simulink model "ASM_Traffic_V2X_Complete_Model_2"  (R2019a)
settings: Solver=ode1  StartTime=SIM.tstart.v  StopTime=Inf  FixedStep=SIM.StepSize.v  RelTol=1e-3
PostLoadFcn:
  | if any(exist('dsrtsu_mdlpostloadfcn', 'file') ~= 0), dsrtsu_mdlpostloadfcn('Execute', bdroot); end
  | try, asm_mdl_postloadfcn(bdroot, 'UpdateModel', 2200); catch, disp(lasterr); end,
undefined symbols (not defined in the file): _SensorPnts_1, _SensorPnts_13, _SensorPnts_17, _SensorPnts_21, _SensorPnts_25, _SensorPnts_29, _SensorPnts_33, _SensorPnts_37, _SensorPnts_41, _SensorPnts_45, _SensorPnts_49, _SensorPnts_5, _SensorPnts_53, _SensorPnts_57, _SensorPnts_9, _to_, CPT, G5A, ITS, MDL, rad, s_to_rpm, SIM
libraries: simulink x169, ASM_VehicleDynamics_lib x126, ASM_Traffic_lib x83, ASM_Utils_lib x49, mdbs x45, ASM_Environment_lib x17, dspindex x12, dsaV2xLibraryAux x10, dsmpblib x6, dsaV2xAsn1Library x4, dsaV2xLibrary x4, ASM_BrakeHydraulics_lib x4
(part 4 of 36)

== system ASM_Traffic_V2X_Complete_Model_2/MDL/MDL_In/Ctrl_ChangeOverValve_1[0_1] ==
  SoftECU : Inport
  RealECU : Inport  Port=2
  Const_Ctrl_ChangeOverValve_1[0_1] : Constant  Value=0
  MultiPortSwitch : MultiPortSwitch  SaturateOnIntegerOverflow=on  InputSameDT=on
  Sw_Ctrl_ChangeOverValve_1[1SoftECU|2RealECU|3Const] : Constant  Value=CPT.MDL_SW.Sw_Ctrl_ChangeOverValve_1.v
  Ctrl_ChangeOverValve_1[0_1] : Outport
  wires:
  MultiPortSwitch/1 -> Ctrl_ChangeOverValve_1[0_1]/1
  Const_Ctrl_ChangeOverValve_1[0_1]/1 -> MultiPortSwitch/4
  RealECU/1 -> MultiPortSwitch/3
  SoftECU/1 -> MultiPortSwitch/2
  Sw_Ctrl_ChangeOverValve_1[1SoftECU|2RealECU|3Const]/1 -> MultiPortSwitch/1

== system ASM_Traffic_V2X_Complete_Model_2/MDL/MDL_In/Ctrl_ChangeOverValve_2[0_1] ==
  SoftECU : Inport
  RealECU : Inport  Port=2
  Const_Ctrl_ChangeOverValve_2[0_1] : Constant  Value=0
  MultiPortSwitch : MultiPortSwitch  SaturateOnIntegerOverflow=on  InputSameDT=on
  Sw_Ctrl_ChangeOverValve_2[1SoftECU|2RealECU|3Const] : Constant  Value=CPT.MDL_SW.Sw_Ctrl_ChangeOverValve_2.v
  Ctrl_ChangeOverValve_2[0_1] : Outport
  wires:
  Sw_Ctrl_ChangeOverValve_2[1SoftECU|2RealECU|3Const]/1 -> MultiPortSwitch/1
  SoftECU/1 -> MultiPortSwitch/2
  RealECU/1 -> MultiPortSwitch/3
  Const_Ctrl_ChangeOverValve_2[0_1]/1 -> MultiPortSwitch/4
  MultiPortSwitch/1 -> Ctrl_ChangeOverValve_2[0_1]/1

== system ASM_Traffic_V2X_Complete_Model_2/MDL/MDL_In/Ctrl_Clutch_4WD[%] ==
  SoftECU : Inport
  RealECU : Inport  Port=2
  Const_Ctrl_Clutch_4WD[%] : Constant  Value=0
  MultiPortSwitch : MultiPortSwitch  SaturateOnIntegerOverflow=on  InputSameDT=on
  Sw_Clutch_4WD[1SoftECU|2RealECU|3Const] : Constant  Value=CPT.MDL_SW.Sw_Clutch_4WD.v
  Ctrl_Clutch_4WD[%] : Outport
  wires:
  Sw_Clutch_4WD[1SoftECU|2RealECU|3Const]/1 -> MultiPortSwitch/1
  SoftECU/1 -> MultiPortSwitch/2
  RealECU/1 -> MultiPortSwitch/3
  Const_Ctrl_Clutch_4WD[%]/1 -> MultiPortSwitch/4
  MultiPortSwitch/1 -> Ctrl_Clutch_4WD[%]/1

== system ASM_Traffic_V2X_Complete_Model_2/MDL/MDL_In/Ctrl_FrontDiff[%] ==
  SoftECU : Inport
  RealECU : Inport  Port=2
  Const_Ctrl_FrontDiff[%] : Constant  Value=0
  MultiPortSwitch : MultiPortSwitch  SaturateOnIntegerOverflow=on  InputSameDT=on
  Sw_Ctrl_FrontDiff[1SoftECU|2RealECU|3Const] : Constant  Value=CPT.MDL_SW.Sw_Ctrl_FrontDiff.v
  Ctrl_FrontDiff[%] : Outport
  wires:
  Sw_Ctrl_FrontDiff[1SoftECU|2RealECU|3Const]/1 -> MultiPortSwitch/1
  SoftECU/1 -> MultiPortSwitch/2
  RealECU/1 -> MultiPortSwitch/3
  Const_Ctrl_FrontDiff[%]/1 -> MultiPortSwitch/4
  MultiPortSwitch/1 -> Ctrl_FrontDiff[%]/1

== system ASM_Traffic_V2X_Complete_Model_2/MDL/MDL_In/Ctrl_HydPump[0_1] ==
  SoftECU : Inport
  RealECU : Inport  Port=2
  Const_Ctrl_HydPump[0_1] : Constant  Value=0
  MultiPortSwitch : MultiPortSwitch  SaturateOnIntegerOverflow=on  InputSameDT=on
  Sw_Ctrl_HydPump[1SoftECU|2RealECU|3Const] : Constant  Value=CPT.MDL_SW.Sw_Ctrl_HydPump.v
  Ctrl_HydPump[0_1] : Outport
  wires:
  Sw_Ctrl_HydPump[1SoftECU|2RealECU|3Const]/1 -> MultiPortSwitch/1
  SoftECU/1 -> MultiPortSwitch/2
  RealECU/1 -> MultiPortSwitch/3
  Const_Ctrl_HydPump[0_1]/1 -> MultiPortSwitch/4
  MultiPortSwitch/1 -> Ctrl_HydPump[0_1]/1

== system ASM_Traffic_V2X_Complete_Model_2/MDL/MDL_In/Ctrl_InletValve_FL[0_1] ==
  SoftECU : Inport
  RealECU : Inport  Port=2
  Const_Ctrl_InletValve_FL[0_1] : Constant  Value=0
  MultiPortSwitch : MultiPortSwitch  SaturateOnIntegerOverflow=on  InputSameDT=on
  Sw_Ctrl_InletValve_FL[1SoftECU|2RealECU|3Const] : Constant  Value=CPT.MDL_SW.Sw_Ctrl_InletValve_FL.v
  Ctrl_InletValve_FL[0_1] : Outport
  wires:
  Sw_Ctrl_InletValve_FL[1SoftECU|2RealECU|3Const]/1 -> MultiPortSwitch/1
  SoftECU/1 -> MultiPortSwitch/2
  RealECU/1 -> MultiPortSwitch/3
  Const_Ctrl_InletValve_FL[0_1]/1 -> MultiPortSwitch/4
  MultiPortSwitch/1 -> Ctrl_InletValve_FL[0_1]/1

== system ASM_Traffic_V2X_Complete_Model_2/MDL/MDL_In/Ctrl_InletValve_FR[0_1] ==
  SoftECU : Inport
  RealECU : Inport  Port=2
  Const_Ctrl_InletValve_FR[0_1] : Constant  Value=0
  MultiPortSwitch : MultiPortSwitch  SaturateOnIntegerOverflow=on  InputSameDT=on
  Sw_Ctrl_InletValve_FR[1SoftECU|2RealECU|3Const] : Constant  Value=CPT.MDL_SW.Sw_Ctrl_InletValve_FR.v
  Ctrl_InletValve_FR[0_1] : Outport
  wires:
  MultiPortSwitch/1 -> Ctrl_InletValve_FR[0_1]/1
  Const_Ctrl_InletValve_FR[0_1]/1 -> MultiPortSwitch/4
  RealECU/1 -> MultiPortSwitch/3
  SoftECU/1 -> MultiPortSwitch/2
  Sw_Ctrl_InletValve_FR[1SoftECU|2RealECU|3Const]/1 -> MultiPortSwitch/1

== system ASM_Traffic_V2X_Complete_Model_2/MDL/MDL_In/Ctrl_InletValve_RL[0_1] ==
  SoftECU : Inport
  RealECU : Inport  Port=2
  Const_Ctrl_InletValve_RL[0_1] : Constant  Value=0
  MultiPortSwitch : MultiPortSwitch  SaturateOnIntegerOverflow=on  InputSameDT=on
  Sw_Ctrl_InletValve_RL[1SoftECU|2RealECU|3Const] : Constant  Value=CPT.MDL_SW.Sw_Ctrl_InletValve_RL.v
  Ctrl_InletValve_RL[0_1] : Outport
  wires:
  MultiPortSwitch/1 -> Ctrl_InletValve_RL[0_1]/1
  Const_Ctrl_InletValve_RL[0_1]/1 -> MultiPortSwitch/4
  RealECU/1 -> MultiPortSwitch/3
  SoftECU/1 -> MultiPortSwitch/2
  Sw_Ctrl_InletValve_RL[1SoftECU|2RealECU|3Const]/1 -> MultiPortSwitch/1

== system ASM_Traffic_V2X_Complete_Model_2/MDL/MDL_In/Ctrl_InletValve_RR[0_1] ==
  SoftECU : Inport
  RealECU : Inport  Port=2
  Const_Ctrl_InletValve_RR[0_1] : Constant  Value=0
  MultiPortSwitch : MultiPortSwitch  SaturateOnIntegerOverflow=on  InputSameDT=on
  Sw_Ctrl_InletValve_RR[1SoftECU|2RealECU|3Const] : Constant  Value=CPT.MDL_SW.Sw_Ctrl_InletValve_RR.v
  Ctrl_InletValve_RR[0_1] : Outport
  wires:
  Sw_Ctrl_InletValve_RR[1SoftECU|2RealECU|3Const]/1 -> MultiPortSwitch/1
  SoftECU/1 -> MultiPortSwitch/2
  RealECU/1 -> MultiPortSwitch/3
  Const_Ctrl_InletValve_RR[0_1]/1 -> MultiPortSwitch/4
  MultiPortSwitch/1 -> Ctrl_InletValve_RR[0_1]/1

== system ASM_Traffic_V2X_Complete_Model_2/MDL/MDL_In/Ctrl_Lockup_Clutch[%] ==
  SoftECU : Inport
  RealECU : Inport  Port=2
  Const_Ctrl_Lockup_Clutch[%] : Constant  Value=0
  MultiPortSwitch : MultiPortSwitch  SaturateOnIntegerOverflow=on  InputSameDT=on
  Sw_Ctrl_Lockup_Clutch[1SoftECU|2RealECU|3Const] : Constant  Value=CPT.MDL_SW.Sw_Ctrl_Lockup_Clutch.v
  Ctrl_Lockup_Clutch[%] : Outport
  wires:
  Sw_Ctrl_Lockup_Clutch[1SoftECU|2RealECU|3Const]/1 -> MultiPortSwitch/1
  SoftECU/1 -> MultiPortSwitch/2
  RealECU/1 -> MultiPortSwitch/3
  Const_Ctrl_Lockup_Clutch[%]/1 -> MultiPortSwitch/4
  MultiPortSwitch/1 -> Ctrl_Lockup_Clutch[%]/1

== system ASM_Traffic_V2X_Complete_Model_2/MDL/MDL_In/Ctrl_OutletValve_FL[0_1] ==
  SoftECU : Inport
  RealECU : Inport  Port=2
  Const_Ctrl_OutletValve_FL[0_1] : Constant  Value=0
  MultiPortSwitch : MultiPortSwitch  SaturateOnIntegerOverflow=on  InputSameDT=on
  Sw_Ctrl_OutletValve_FL[1SoftECU|2RealECU|3Const] : Constant  Value=CPT.MDL_SW.Sw_Ctrl_OutletValve_FL.v
  Ctrl_OutletValve_FL[0_1] : Outport
  wires:
  Sw_Ctrl_OutletValve_FL[1SoftECU|2RealECU|3Const]/1 -> MultiPortSwitch/1
  SoftECU/1 -> MultiPortSwitch/2
  RealECU/1 -> MultiPortSwitch/3
  Const_Ctrl_OutletValve_FL[0_1]/1 -> MultiPortSwitch/4
  MultiPortSwitch/1 -> Ctrl_OutletValve_FL[0_1]/1

== system ASM_Traffic_V2X_Complete_Model_2/MDL/MDL_In/Ctrl_OutletValve_FR[0_1] ==
  SoftECU : Inport
  RealECU : Inport  Port=2
  Const_Ctrl_OutletValve_FR[0_1] : Constant  Value=0
  MultiPortSwitch : MultiPortSwitch  SaturateOnIntegerOverflow=on  InputSameDT=on
  Sw_Ctrl_OutletValve_FR[1SoftECU|2RealECU|3Const] : Constant  Value=CPT.MDL_SW.Sw_Ctrl_OutletValve_FR.v
  Ctrl_OutletValve_FR[0_1] : Outport
  wires:
  MultiPortSwitch/1 -> Ctrl_OutletValve_FR[0_1]/1
  Const_Ctrl_OutletValve_FR[0_1]/1 -> MultiPortSwitch/4
  RealECU/1 -> MultiPortSwitch/3
  SoftECU/1 -> MultiPortSwitch/2
  Sw_Ctrl_OutletValve_FR[1SoftECU|2RealECU|3Const]/1 -> MultiPortSwitch/1

== system ASM_Traffic_V2X_Complete_Model_2/MDL/MDL_In/Ctrl_OutletValve_RL[0_1] ==
  SoftECU : Inport
  RealECU : Inport  Port=2
  Const_Ctrl_OutletValve_RL[0_1] : Constant  Value=0
  MultiPortSwitch : MultiPortSwitch  SaturateOnIntegerOverflow=on  InputSameDT=on
  Sw_Ctrl_OutletValve_RL[1SoftECU|2RealECU|3Const] : Constant  Value=CPT.MDL_SW.Sw_Ctrl_OutletValve_RL.v
  Ctrl_OutletValve_RL[0_1] : Outport
  wires:
  MultiPortSwitch/1 -> Ctrl_OutletValve_RL[0_1]/1
  Const_Ctrl_OutletValve_RL[0_1]/1 -> MultiPortSwitch/4
  RealECU/1 -> MultiPortSwitch/3
  SoftECU/1 -> MultiPortSwitch/2
  Sw_Ctrl_OutletValve_RL[1SoftECU|2RealECU|3Const]/1 -> MultiPortSwitch/1

== system ASM_Traffic_V2X_Complete_Model_2/MDL/MDL_In/Ctrl_OutletValve_RR[0_1] ==
  SoftECU : Inport
  RealECU : Inport  Port=2
  Const_Ctrl_OutletValve_RR[0_1] : Constant  Value=0
  MultiPortSwitch : MultiPortSwitch  SaturateOnIntegerOverflow=on  InputSameDT=on
  Sw_Ctrl_OutletValve_RR[1SoftECU|2RealECU|3Const] : Constant  Value=CPT.MDL_SW.Sw_Ctrl_OutletValve_RR.v
  Ctrl_OutletValve_RR[0_1] : Outport
  wires:
  Sw_Ctrl_OutletValve_RR[1SoftECU|2RealECU|3Const]/1 -> MultiPortSwitch/1
  SoftECU/1 -> MultiPortSwitch/2
  RealECU/1 -> MultiPortSwitch/3
  Const_Ctrl_OutletValve_RR[0_1]/1 -> MultiPortSwitch/4
  MultiPortSwitch/1 -> Ctrl_OutletValve_RR[0_1]/1

== system ASM_Traffic_V2X_Complete_Model_2/MDL/MDL_In/Ctrl_Parking_Pawl[0|1] ==
  SoftECU : Inport
  RealECU : Inport  Port=2
  Const_Park_Lock[0|1] : Constant  Value=0
  MultiPortSwitch : MultiPortSwitch  SaturateOnIntegerOverflow=on  InputSameDT=on
  Sw_Parking_Pawl[1SoftECU|2RealECU|3Const] : Constant  Value=CPT.MDL_SW.Sw_Parking_Pawl.v
  Ctrl_Parking_Pawl[0|1] : Outport
  wires:
  Sw_Parking_Pawl[1SoftECU|2RealECU|3Const]/1 -> MultiPortSwitch/1
  SoftECU/1 -> MultiPortSwitch/2
  RealECU/1 -> MultiPortSwitch/3
  Const_Park_Lock[0|1]/1 -> MultiPortSwitch/4
  MultiPortSwitch/1 -> Ctrl_Parking_Pawl[0|1]/1

== system ASM_Traffic_V2X_Complete_Model_2/MDL/MDL_In/Ctrl_PreChargeValve_1[0_1] ==
  SoftECU : Inport
  RealECU : Inport  Port=2
  Const_Ctrl_PreChargeValve_1[0_1] : Constant  Value=0
  MultiPortSwitch : MultiPortSwitch  SaturateOnIntegerOverflow=on  InputSameDT=on
  Sw_Ctrl_PreChargeValve_1[1SoftECU|2RealECU|3Const] : Constant  Value=CPT.MDL_SW.Sw_Ctrl_PreChargeValve_1.v
  Ctrl_PreChargeValve_1[0_1] : Outport
  wires:
  Sw_Ctrl_PreChargeValve_1[1SoftECU|2RealECU|3Const]/1 -> MultiPortSwitch/1
  SoftECU/1 -> MultiPortSwitch/2
  RealECU/1 -> MultiPortSwitch/3
  Const_Ctrl_PreChargeValve_1[0_1]/1 -> MultiPortSwitch/4
  MultiPortSwitch/1 -> Ctrl_PreChargeValve_1[0_1]/1

== system ASM_Traffic_V2X_Complete_Model_2/MDL/MDL_In/Ctrl_PreChargeValve_2[0_1] ==
  SoftECU : Inport
  RealECU : Inport  Port=2
  Const_Ctrl_PreChargeValve_2[0_1] : Constant  Value=0
  MultiPortSwitch : MultiPortSwitch  SaturateOnIntegerOverflow=on  InputSameDT=on
  Sw_Ctrl_PreChargeValve_2[1SoftECU|2RealECU|3Const] : Constant  Value=CPT.MDL_SW.Sw_Ctrl_PreChargeValve_2.v
  Ctrl_PreChargeValve_2[0_1] : Outport
  wires:
  MultiPortSwitch/1 -> Ctrl_PreChargeValve_2[0_1]/1
  Const_Ctrl_PreChargeValve_2[0_1]/1 -> MultiPortSwitch/4
  RealECU/1 -> MultiPortSwitch/3
  SoftECU/1 -> MultiPortSwitch/2
  Sw_Ctrl_PreChargeValve_2[1SoftECU|2RealECU|3Const]/1 -> MultiPortSwitch/1

== system ASM_Traffic_V2X_Complete_Model_2/MDL/MDL_In/Ctrl_RearDiff[%] ==
  SoftECU : Inport
  RealECU : Inport  Port=2
  Const_Ctrl_RearDiff[%] : Constant  Value=0
  MultiPortSwitch : MultiPortSwitch  SaturateOnIntegerOverflow=on  InputSameDT=on
  Sw_Ctrl_RearDiff[1SoftECU|2RealECU|3Const] : Constant  Value=CPT.MDL_SW.Sw_Ctrl_RearDiff.v
  Ctrl_RearDiff[%] : Outport
  wires:
  MultiPortSwitch/1 -> Ctrl_RearDiff[%]/1
  Const_Ctrl_RearDiff[%]/1 -> MultiPortSwitch/4
  RealECU/1 -> MultiPortSwitch/3
  SoftECU/1 -> MultiPortSwitch/2
  Sw_Ctrl_RearDiff[1SoftECU|2RealECU|3Const]/1 -> MultiPortSwitch/1

== system ASM_Traffic_V2X_Complete_Model_2/MDL/MDL_In/Displ_SteeringRod[Displ;Displ_dt][m;m|s] ==
  SoftECU : Inport
  RealECU : Inport  Port=2
  Const_Displ_SteeringRod[Displ;Displ_dt][m;m|s] : Constant  Value=[0;0]
  MultiPortSwitch : MultiPortSwitch  SaturateOnIntegerOverflow=on  InputSameDT=on
  Sw_Displ_SteeringRod[1SoftECU|2RealECU|3Const] : Constant  Value=CPT.MDL_SW.Sw_Displ_SteeringRod.v
  Displ_SteeringRod[Displ;Displ_dt][m;m|s] : Outport
  wires:
  Sw_Displ_SteeringRod[1SoftECU|2RealECU|3Const]/1 -> MultiPortSwitch/1
  SoftECU/1 -> MultiPortSwitch/2
  RealECU/1 -> MultiPortSwitch/3
  Const_Displ_SteeringRod[Displ;Displ_dt][m;m|s]/1 -> MultiPortSwitch/4
  MultiPortSwitch/1 -> Displ_SteeringRod[Displ;Displ_dt][m;m|s]/1

== system ASM_Traffic_V2X_Complete_Model_2/MDL/MDL_In/ECU_ESP_Mode[0None|1ABS|2ESP|3ASR] ==
  SoftECU : Inport
  RealECU : Inport  Port=2
  Const_ECU_ESP_Mode[0None|1ABS|2ESP|3ASR] : Constant  Value=0
  MultiPortSwitch : MultiPortSwitch  SaturateOnIntegerOverflow=on  InputSameDT=on
  Sw_ECU_Mode[1SoftECU|2RealECU|3Const] : Constant  Value=CPT.MDL_SW.Sw_ECU_ESP_Mode.v
  ECU_ESP_Mode[0None|1ABS|2ESP|3ASR] : Outport
  wires:
  MultiPortSwitch/1 -> ECU_ESP_Mode[0None|1ABS|2ESP|3ASR]/1
  Const_ECU_ESP_Mode[0None|1ABS|2ESP|3ASR]/1 -> MultiPortSwitch/4
  RealECU/1 -> MultiPortSwitch/3
  SoftECU/1 -> MultiPortSwitch/2
  Sw_ECU_Mode[1SoftECU|2RealECU|3Const]/1 -> MultiPortSwitch/1

== system ASM_Traffic_V2X_Complete_Model_2/MDL/MDL_In/EPSMotorStates_External[Angle;Angle_dt][rad;rad|s] ==
  SoftECU : Inport
  RealECU : Inport  Port=2
  Const_EPSMotorStates_External[Angle;Angle_dt][rad;rad|s] : Constant  Value=[0;0]
  MultiPortSwitch : MultiPortSwitch  SaturateOnIntegerOverflow=on  InputSameDT=on
  Sw_EPSMotorStates_External[1SoftECU|2RealECU|3Const] : Constant  Value=CPT.MDL_SW.Sw_EPSMotorStates_External.v
  EPSMotorStates_External[Angle;Angle_dt][rad;rad|s] : Outport
  wires:
  MultiPortSwitch/1 -> EPSMotorStates_External[Angle;Angle_dt][rad;rad|s]/1
  Const_EPSMotorStates_External[Angle;Angle_dt][rad;rad|s]/1 -> MultiPortSwitch/4
  RealECU/1 -> MultiPortSwitch/3
  SoftECU/1 -> MultiPortSwitch/2
  Sw_EPSMotorStates_External[1SoftECU|2RealECU|3Const]/1 -> MultiPortSwitch/1

== system ASM_Traffic_V2X_Complete_Model_2/MDL/MDL_In/Enable_TrqDecrease_Fast_ESP[0|1] ==
  SoftECU : Inport
  RealECU : Inport  Port=2
  Const_Enable_TrqDecrease_Fast[0|1] : Constant  Value=0
  MultiPortSwitch : MultiPortSwitch  SaturateOnIntegerOverflow=on  InputSameDT=on
  Sw_Enable_TrqDecrease_Fast[1SoftECU|2RealECU|3Const] : Constant  Value=CPT.MDL_SW.Sw_Enable_TrqDecrease_Fast_ESP.v
  Enable_TrqDecrease_Fast[0|1] : Outport
  wires:
  Sw_Enable_TrqDecrease_Fast[1SoftECU|2RealECU|3Const]/1 -> MultiPortSwitch/1
  SoftECU/1 -> MultiPortSwitch/2
  RealECU/1 -> MultiPortSwitch/3
  Const_Enable_TrqDecrease_Fast[0|1]/1 -> MultiPortSwitch/4
  MultiPortSwitch/1 -> Enable_TrqDecrease_Fast[0|1]/1

== system ASM_Traffic_V2X_Complete_Model_2/MDL/MDL_In/Enable_TrqDecrease_Slow_ESP[0|1] ==
  SoftECU : Inport
  RealECU : Inport  Port=2
  Const_Enable_TrqDecrease_Slow[0|1] : Constant  Value=0
  MultiPortSwitch : MultiPortSwitch  SaturateOnIntegerOverflow=on  InputSameDT=on
  Sw_Enable_TrqDecrease_Slow[1SoftECU|2RealECU|3Const] : Constant  Value=CPT.MDL_SW.Sw_Enable_TrqDecrease_Slow_ESP.v
  Enable_TrqDecrease_Slow[0|1] : Outport
  wires:
  Sw_Enable_TrqDecrease_Slow[1SoftECU|2RealECU|3Const]/1 -> MultiPortSwitch/1
  SoftECU/1 -> MultiPortSwitch/2
  RealECU/1 -> MultiPortSwitch/3
  Const_Enable_TrqDecrease_Slow[0|1]/1 -> MultiPortSwitch/4
  MultiPortSwitch/1 -> Enable_TrqDecrease_Slow[0|1]/1

== system ASM_Traffic_V2X_Complete_Model_2/MDL/MDL_In/Enable_TrqIncrease_ESP[0|1] ==
  SoftECU : Inport
  RealECU : Inport  Port=2
  Const_Enable_TrqIncrease[0|1] : Constant  Value=0
  MultiPortSwitch : MultiPortSwitch  SaturateOnIntegerOverflow=on  InputSameDT=on
  Sw_Enable_TrqIncrease[1SoftECU|2RealECU|3Const] : Constant  Value=CPT.MDL_SW.Sw_Enable_TrqIncrease_ESP.v
  Enable_TrqIncrease[0|1] : Outport
  wires:
  Sw_Enable_TrqIncrease[1SoftECU|2RealECU|3Const]/1 -> MultiPortSwitch/1
  SoftECU/1 -> MultiPortSwitch/2
  RealECU/1 -> MultiPortSwitch/3
  Const_Enable_TrqIncrease[0|1]/1 -> MultiPortSwitch/4
  MultiPortSwitch/1 -> Enable_TrqIncrease[0|1]/1

== system ASM_Traffic_V2X_Complete_Model_2/MDL/MDL_In/Enable_Trq_Decrease_ACC[0|1] ==
  SoftECU : Inport
  RealECU : Inport  Port=2
  Const_Enable_Trq_Decrease_ACC[0|1] : Constant  Value=0
  MultiPortSwitch : MultiPortSwitch  SaturateOnIntegerOverflow=on  InputSameDT=on
  Sw_Enable_Trq_Decrease_ACC[1SoftECU|2RealECU|3Const] : Constant  Value=CPT.MDL_SW.Sw_Enable_Trq_Decrease_ACC.v
  Ctrl_ChangeOverValve_2[0|1] : Outport
  wires:
  Sw_Enable_Trq_Decrease_ACC[1SoftECU|2RealECU|3Const]/1 -> MultiPortSwitch/1
  SoftECU/1 -> MultiPortSwitch/2
  RealECU/1 -> MultiPortSwitch/3
  Const_Enable_Trq_Decrease_ACC[0|1]/1 -> MultiPortSwitch/4
  MultiPortSwitch/1 -> Ctrl_ChangeOverValve_2[0|1]/1

== system ASM_Traffic_V2X_Complete_Model_2/MDL/MDL_In/Enable_Trq_Increase_ACC[0|1] ==
  SoftECU : Inport
  RealECU : Inport  Port=2
  Const_Enable_Trq_Increase_ACC[0|1] : Constant  Value=0
  MultiPortSwitch : MultiPortSwitch  SaturateOnIntegerOverflow=on  InputSameDT=on
  Sw_Enable_Trq_Increase_ACC[1SoftECU|2RealECU|3Const] : Constant  Value=CPT.MDL_SW.Sw_Enable_Trq_Increase_ACC.v
  Enable_Trq_Increase_ACC[0|1] : Outport
  wires:
  MultiPortSwitch/1 -> Enable_Trq_Increase_ACC[0|1]/1
  Const_Enable_Trq_Increase_ACC[0|1]/1 -> MultiPortSwitch/4
  RealECU/1 -> MultiPortSwitch/3
  SoftECU/1 -> MultiPortSwitch/2
  Sw_Enable_Trq_Increase_ACC[1SoftECU|2RealECU|3Const]/1 -> MultiPortSwitch/1

== system ASM_Traffic_V2X_Complete_Model_2/MDL/MDL_In/Enable_p_Brake_Desired[0|1] ==
  SoftECU : Inport
  RealECU : Inport  Port=2
  Const_Enable_p_Brake_Desired[0|1] : Constant  Value=0
  MultiPortSwitch : MultiPortSwitch  SaturateOnIntegerOverflow=on  InputSameDT=on
  Sw_Enable_p_Brake_Desired[1SoftECU|2RealECU|3Const] : Constant  Value=CPT.MDL_SW.Sw_Enable_p_Brake_Desired.v
  Enable_p_Brake_Desired[0|1] : Outport
  wires:
  MultiPortSwitch/1 -> Enable_p_Brake_Desired[0|1]/1
  Const_Enable_p_Brake_Desired[0|1]/1 -> MultiPortSwitch/4
  RealECU/1 -> MultiPortSwitch/3
  SoftECU/1 -> MultiPortSwitch/2
  Sw_Enable_p_Brake_Desired[1SoftECU|2RealECU|3Const]/1 -> MultiPortSwitch/1

== system ASM_Traffic_V2X_Complete_Model_2/MDL/MDL_In/Engine_Dynamic_Fast[0|1] ==
  SoftECU : Inport
  RealECU : Inport  Port=2
  Const_Engine_Dynamic_Fast[0|1]] : Constant  Value=0
  Engine_Dynamic_Fast[0|1][1SoftECU|2RealECU|3Const] : Constant  Value=CPT.MDL_SW.Sw_Engine_Dynamic_Fast.v
  MultiPortSwitch : MultiPortSwitch  SaturateOnIntegerOverflow=on  InputSameDT=on
  Engine_Dynamic_Fast[0|1] : Outport
  wires:
  MultiPortSwitch/1 -> Engine_Dynamic_Fast[0|1]/1
  Const_Engine_Dynamic_Fast[0|1]]/1 -> MultiPortSwitch/4
  RealECU/1 -> MultiPortSwitch/3
  SoftECU/1 -> MultiPortSwitch/2
  Engine_Dynamic_Fast[0|1][1SoftECU|2RealECU|3Const]/1 -> MultiPortSwitch/1

== system ASM_Traffic_V2X_Complete_Model_2/MDL/MDL_In/Factor_Trq_Engine_Red[%] ==
  SoftECU : Inport
  RealECU : Inport  Port=2
  Const_Factor_Trq_Engine_Red[%] : Constant  Value=0
  MultiPortSwitch : MultiPortSwitch  SaturateOnIntegerOverflow=on  InputSameDT=on
  Sw_Factor_Trq_Engine_Red[1SoftECU|2RealECU|3Const] : Constant  Value=CPT.MDL_SW.Sw_Factor_Trq_Engine_Red.v
  Factor_Trq_Engine_Red[%] : Outport
  wires:
  MultiPortSwitch/1 -> Factor_Trq_Engine_Red[%]/1
  Const_Factor_Trq_Engine_Red[%]/1 -> MultiPortSwitch/4
  RealECU/1 -> MultiPortSwitch/3
  SoftECU/1 -> MultiPortSwitch/2
  Sw_Factor_Trq_Engine_Red[1SoftECU|2RealECU|3Const]/1 -> MultiPortSwitch/1

== system ASM_Traffic_V2X_Complete_Model_2/MDL/MDL_In/Gear[] ==
  SoftECU : Inport
  RealECU : Inport  Port=2
  Const_Gear[] : Constant  Value=0
  MultiPortSwitch : MultiPortSwitch  SaturateOnIntegerOverflow=on  InputSameDT=on
  Sw_Gear[1SoftECU|2RealECU|3Const] : Constant  Value=CPT.MDL_SW.Sw_Gear.v
  Gear[] : Outport
  wires:
  MultiPortSwitch/1 -> Gear[]/1
  Const_Gear[]/1 -> MultiPortSwitch/4
  RealECU/1 -> MultiPortSwitch/3
  SoftECU/1 -> MultiPortSwitch/2
  Sw_Gear[1SoftECU|2RealECU|3Const]/1 -> MultiPortSwitch/1

== system ASM_Traffic_V2X_Complete_Model_2/MDL/MDL_In/Pos_AccPedal_Driver_Des[%] ==
  SoftECU : Inport
  RealECU : Inport  Port=2
  Const_Pos_AccPedal_Driver_Des[%] : Constant  Value=0
  MultiPortSwitch : MultiPortSwitch  SaturateOnIntegerOverflow=on  InputSameDT=on
  Sw_Pos_AccPedal_Driver_Des[1SoftECU|2RealECU|3Const] : Constant  Value=CPT.MDL_SW.Sw_Pos_AccPedal_Driver_Des.v
  Pos_AccPedal_Driver_Des[%] : Outport
  wires:
  Sw_Pos_AccPedal_Driver_Des[1SoftECU|2RealECU|3Const]/1 -> MultiPortSwitch/1
  SoftECU/1 -> MultiPortSwitch/2
  RealECU/1 -> MultiPortSwitch/3
  Const_Pos_AccPedal_Driver_Des[%]/1 -> MultiPortSwitch/4
  MultiPortSwitch/1 -> Pos_AccPedal_Driver_Des[%]/1

== system ASM_Traffic_V2X_Complete_Model_2/MDL/MDL_In/Pos_AccPedal_Influenced[%] ==
  SoftECU : Inport
  RealECU : Inport  Port=2
  Const_Pos_AccPedal_Influenced[%] : Constant  Value=0
  MultiPortSwitch : MultiPortSwitch  SaturateOnIntegerOverflow=on  InputSameDT=on
  Sw_Pos_AccPedal_Influenced[1SoftECU|2RealECU|3Const] : Constant  Value=CPT.MDL_SW.Sw_Pos_AccPedal_Influenced.v
  Pos_AccPedal_Influenced[%] : Outport
  wires:
  Sw_Pos_AccPedal_Influenced[1SoftECU|2RealECU|3Const]/1 -> MultiPortSwitch/1
  SoftECU/1 -> MultiPortSwitch/2
  RealECU/1 -> MultiPortSwitch/3
  Const_Pos_AccPedal_Influenced[%]/1 -> MultiPortSwitch/4
  MultiPortSwitch/1 -> Pos_AccPedal_Influenced[%]/1

== system ASM_Traffic_V2X_Complete_Model_2/MDL/MDL_In/State_Engine[0|1|2|3|4] ==
  SoftECU : Inport
  RealECU : Inport  Port=2
  Const_State_Engine[0|1|2|3|4] : Constant  Value=0
  MultiPortSwitch : MultiPortSwitch  SaturateOnIntegerOverflow=on  InputSameDT=on
  Sw_State_Engine[1SoftECU|2RealECU|3Const] : Constant  Value=CPT.MDL_SW.Sw_State_Engine.v
  State_Engine[0|1|2|3|4] : Outport
  wires:
  RealECU/1 -> MultiPortSwitch/3
  SoftECU/1 -> MultiPortSwitch/2
  Sw_State_Engine[1SoftECU|2RealECU|3Const]/1 -> MultiPortSwitch/1
  MultiPortSwitch/1 -> State_Engine[0|1|2|3|4]/1
  Const_State_Engine[0|1|2|3|4]/1 -> MultiPortSwitch/4

== system ASM_Traffic_V2X_Complete_Model_2/MDL/MDL_In/Sw_AC[0|1] ==
  SoftECU : Inport
  RealECU : Inport  Port=2
  Const_Sw_AC[0|1] : Constant  Value=0
  MultiPortSwitch : MultiPortSwitch  SaturateOnIntegerOverflow=on  InputSameDT=on
  Sw_Ctrl_AC[1SoftECU|2RealECU|3Const] : Constant  Value=CPT.MDL_SW.Sw_Sw_AC.v
  Sw_AC[0|1] : Outport
  wires:
  Sw_Ctrl_AC[1SoftECU|2RealECU|3Const]/1 -> MultiPortSwitch/1
  SoftECU/1 -> MultiPortSwitch/2
  RealECU/1 -> MultiPortSwitch/3
  Const_Sw_AC[0|1]/1 -> MultiPortSwitch/4
  MultiPortSwitch/1 -> Sw_AC[0|1]/1

== system ASM_Traffic_V2X_Complete_Model_2/MDL/MDL_In/Sw_Ignition[0|1] ==
  SoftECU : Inport
  RealECU : Inport  Port=2
  Const_Sw_Ignition[0|1] : Constant  Value=0
  MultiPortSwitch : MultiPortSwitch  SaturateOnIntegerOverflow=on  InputSameDT=on
  Sw_Ignition[1SoftECU|2RealECU|3Const] : Constant  Value=CPT.MDL_SW.Sw_Ignition.v
  Sw_Ignition[0|1] : Outport
  wires:
  Sw_Ignition[1SoftECU|2RealECU|3Const]/1 -> MultiPortSwitch/1
  SoftECU/1 -> MultiPortSwitch/2
  RealECU/1 -> MultiPortSwitch/3
  Const_Sw_Ignition[0|1]/1 -> MultiPortSwitch/4
  MultiPortSwitch/1 -> Sw_Ignition[0|1]/1

== system ASM_Traffic_V2X_Complete_Model_2/MDL/MDL_In/Sw_StarterReq[0|1] ==
  SoftECU : Inport
  RealECU : Inport  Port=2
  Const_Sw_StarterReq[0|1] : Constant  Value=0
  MultiPortSwitch : MultiPortSwitch  SaturateOnIntegerOverflow=on  InputSameDT=on
  Sw_StarterReq[1SoftECU|2RealECU|3Const] : Constant  Value=CPT.MDL_SW.Sw_StarterReq.v
  Sw_StarterReq[0|1] : Outport
  wires:
  MultiPortSwitch/1 -> Sw_StarterReq[0|1]/1
  Const_Sw_StarterReq[0|1]/1 -> MultiPortSwitch/4
  RealECU/1 -> MultiPortSwitch/3
  SoftECU/1 -> MultiPortSwitch/2
  Sw_StarterReq[1SoftECU|2RealECU|3Const]/1 -> MultiPortSwitch/1

== system ASM_Traffic_V2X_Complete_Model_2/MDL/MDL_In/Sw_Starter[0Off|1On] ==
  SoftECU : Inport
  RealECU : Inport  Port=2
  Const_Sw_Starter[0Off|1On] : Constant  Value=0
  MultiPortSwitch : MultiPortSwitch  SaturateOnIntegerOverflow=on  InputSameDT=on
  Sw_Starter[1SoftECU|2RealECU|3Const] : Constant  Value=CPT.MDL_SW.Sw_Starter.v
  Sw_Starter[0Off|1On] : Outport
  wires:
  MultiPortSwitch/1 -> Sw_Starter[0Off|1On]/1
  Const_Sw_Starter[0Off|1On]/1 -> MultiPortSwitch/4
  RealECU/1 -> MultiPortSwitch/3
  SoftECU/1 -> MultiPortSwitch/2
  Sw_Starter[1SoftECU|2RealECU|3Const]/1 -> MultiPortSwitch/1

== system ASM_Traffic_V2X_Complete_Model_2/MDL/MDL_In/Trq_DecreaseRequest_ACC[Nm] ==
  SoftECU : Inport
  RealECU : Inport  Port=2
  Const_Trq_DecreaseRequest_ACC[Nm] : Constant  Value=0
  MultiPortSwitch : MultiPortSwitch  SaturateOnIntegerOverflow=on  InputSameDT=on
  Sw_Trq_DecreaseRequest_ACC[1SoftECU|2RealECU|3Const] : Constant  Value=CPT.MDL_SW.Sw_Trq_DecreaseRequest_ACC.v
  Trq_DecreaseRequest_ACC[Nm] : Outport
  wires:
  Sw_Trq_DecreaseRequest_ACC[1SoftECU|2RealECU|3Const]/1 -> MultiPortSwitch/1
  SoftECU/1 -> MultiPortSwitch/2
  RealECU/1 -> MultiPortSwitch/3
  Const_Trq_DecreaseRequest_ACC[Nm]/1 -> MultiPortSwitch/4
  MultiPortSwitch/1 -> Trq_DecreaseRequest_ACC[Nm]/1

== system ASM_Traffic_V2X_Complete_Model_2/MDL/MDL_In/Trq_DecreaseRequest_Fast_ESP[Nm] ==
  SoftECU : Inport
  RealECU : Inport  Port=2
  Const_Trq_DecreaseRequest_Fast[Nm] : Constant  Value=0
  MultiPortSwitch : MultiPortSwitch  SaturateOnIntegerOverflow=on  InputSameDT=on
  Sw_Trq_DecreaseRequest_Fast[1SoftECU|2RealECU|3Const] : Constant  Value=CPT.MDL_SW.Sw_Trq_DecreaseRequest_Fast_ESP.v
  Trq_DecreaseRequest_Fast[Nm] : Outport
  wires:
  MultiPortSwitch/1 -> Trq_DecreaseRequest_Fast[Nm]/1
  Const_Trq_DecreaseRequest_Fast[Nm]/1 -> MultiPortSwitch/4
  RealECU/1 -> MultiPortSwitch/3
  SoftECU/1 -> MultiPortSwitch/2
  Sw_Trq_DecreaseRequest_Fast[1SoftECU|2RealECU|3Const]/1 -> MultiPortSwitch/1

== system ASM_Traffic_V2X_Complete_Model_2/MDL/MDL_In/Trq_DecreaseRequest_Slow_ESP[Nm] ==
  SoftECU : Inport
  RealECU : Inport  Port=2
  Const_Trq_DecreaseRequest_Slow[Nm] : Constant  Value=0
  MultiPortSwitch : MultiPortSwitch  SaturateOnIntegerOverflow=on  InputSameDT=on
  Sw_Trq_DecreaseRequest_Slow[1SoftECU|2RealECU|3Const] : Constant  Value=CPT.MDL_SW.Sw_Trq_DecreaseRequest_Slow_ESP.v
  Trq_DecreaseRequest_Slow[Nm] : Outport
  wires:
  MultiPortSwitch/1 -> Trq_DecreaseRequest_Slow[Nm]/1
  Const_Trq_DecreaseRequest_Slow[Nm]/1 -> MultiPortSwitch/4
  RealECU/1 -> MultiPortSwitch/3
  SoftECU/1 -> MultiPortSwitch/2
  Sw_Trq_DecreaseRequest_Slow[1SoftECU|2RealECU|3Const]/1 -> MultiPortSwitch/1

== system ASM_Traffic_V2X_Complete_Model_2/MDL/MDL_In/Trq_IncreaseRequest_ACC[Nm]2 ==
  SoftECU : Inport
  RealECU : Inport  Port=2
  Const_Trq_IncreaseRequest_ACC[Nm] : Constant  Value=0
  MultiPortSwitch : MultiPortSwitch  SaturateOnIntegerOverflow=on  InputSameDT=on
  Sw_Trq_IncreaseRequest_ACC[1SoftECU|2RealECU|3Const] : Constant  Value=CPT.MDL_SW.Sw_Trq_IncreaseRequest_ACC.v
  Trq_IncreaseRequest_ACC[Nm] : Outport
  wires:
  MultiPortSwitch/1 -> Trq_IncreaseRequest_ACC[Nm]/1
  Const_Trq_IncreaseRequest_ACC[Nm]/1 -> MultiPortSwitch/4
  RealECU/1 -> MultiPortSwitch/3
  SoftECU/1 -> MultiPortSwitch/2
  Sw_Trq_IncreaseRequest_ACC[1SoftECU|2RealECU|3Const]/1 -> MultiPortSwitch/1

== system ASM_Traffic_V2X_Complete_Model_2/MDL/MDL_In/Trq_IncreaseRequest_ESP[Nm] ==
  SoftECU : Inport
  RealECU : Inport  Port=2
  Const_Trq_IncreaseRequest[Nm] : Constant  Value=0
  MultiPortSwitch : MultiPortSwitch  SaturateOnIntegerOverflow=on  InputSameDT=on
  Sw_Trq_IncreaseRequest[1SoftECU|2RealECU|3Const] : Constant  Value=CPT.MDL_SW.Sw_Trq_IncreaseRequest_ESP.v
  Trq_IncreaseRequest[Nm] : Outport
  wires:
  MultiPortSwitch/1 -> Trq_IncreaseRequest[Nm]/1
  Const_Trq_IncreaseRequest[Nm]/1 -> MultiPortSwitch/4
  RealECU/1 -> MultiPortSwitch/3
  SoftECU/1 -> MultiPortSwitch/2
  Sw_Trq_IncreaseRequest[1SoftECU|2RealECU|3Const]/1 -> MultiPortSwitch/1

== system ASM_Traffic_V2X_Complete_Model_2/MDL/MDL_In/Trq_PowerSteering[Nm] ==
  SoftECU : Inport
  RealECU : Inport  Port=2
  Const_Trq_PowerSteering[Nm] : Constant  Value=0
  MultiPortSwitch : MultiPortSwitch  SaturateOnIntegerOverflow=on  InputSameDT=on
  Sw_PowerSteering[1SoftECU|2RealECU|3Const] : Constant  Value=CPT.MDL_SW.Sw_PowerSteering.v
  Trq_PowerSteering[Nm] : Outport
  wires:
  MultiPortSwitch/1 -> Trq_PowerSteering[Nm]/1
  Const_Trq_PowerSteering[Nm]/1 -> MultiPortSwitch/4
  RealECU/1 -> MultiPortSwitch/3
  SoftECU/1 -> MultiPortSwitch/2
  Sw_PowerSteering[1SoftECU|2RealECU|3Const]/1 -> MultiPortSwitch/1

== system ASM_Traffic_V2X_Complete_Model_2/MDL/MDL_In/p_Brake_Desired[bar] ==
  SoftECU : Inport
  RealECU : Inport  Port=2
  Const_p_Brake_Desired[bar] : Constant  Value=0
  MultiPortSwitch : MultiPortSwitch  SaturateOnIntegerOverflow=on  InputSameDT=on
  Sw_p_Brake_Desired[1SoftECU|2RealECU|3Const] : Constant  Value=CPT.MDL_SW.Sw_p_Brake_Desired.v
  p_Brake_Desired[bar] : Outport
  wires:
  Sw_p_Brake_Desired[1SoftECU|2RealECU|3Const]/1 -> MultiPortSwitch/1
  SoftECU/1 -> MultiPortSwitch/2
  RealECU/1 -> MultiPortSwitch/3
  Const_p_Brake_Desired[bar]/1 -> MultiPortSwitch/4
  MultiPortSwitch/1 -> p_Brake_Desired[bar]/1

== system ASM_Traffic_V2X_Complete_Model_2/MDL/SoftECU/ASMSignalCollector ==
  BusCreator : BusCreator  Inputs=6
  ChangeLabel : Subsystem
      mask Display: disp('')
  tag scope: ASMBUS_SoftECU=global
  wires:
  ChangeLabel/1(Out) -> BusCreator/6
  [ASMBUS_SoftECU_StartButton] -> ChangeLabel/1(In)
  [ASMBUS_SoftECU_PowerSteering] -> BusCreator/5
  BusCreator/1 -> [ASMBUS_SoftECU]  "SoftECU"
  [ASMBUS_SoftECU_Engine] -> BusCreator/1
  [ASMBUS_SoftECU_Brake] -> BusCreator/2
  [ASMBUS_SoftECU_ACC] -> BusCreator/3
  [ASMBUS_SoftECU_Transmission] -> BusCreator/4

== system ASM_Traffic_V2X_Complete_Model_2/MDL/SoftECU/DisableReset ==
  note: Start button is not reset, if crankshaft reset is disabled
  Reset_VehicleStates[0|1] : Inport
  MultiPortSwitch : MultiPortSwitch  DataPortOrder=Zero-based contiguous  Inputs=2  zeroidx=on  SaturateOnIntegerOverflow=on  InputSameDT=on
  NO_Reset : Constant  Value=0
  Reset[0|1] : Outport
  wires:
  Reset_VehicleStates[0|1]/1 -> MultiPortSwitch/3
  NO_Reset/1 -> MultiPortSwitch/2
  [TAG_Drivetrain_Sw_CrankShaft_Reset] -> MultiPortSwitch/1
  MultiPortSwitch/1 -> Reset[0|1]/1

== system ASM_Traffic_V2X_Complete_Model_2/MDL/SoftECU/Map_Inputs ==
  Reset[0|1] : Inport
  ECU_Commands[] : Inport  Port=2
  Switches_ESP_User : Inport  Port=3
  Bus Selector2 : BusSelector  OutputSignals=Sw_ESP_Control_Mode[1ManSched|2Manual],Sw_ESP[0Off|1ABS|2ESP],SW_ASR[0Off|1On]
  Maneuver : Subsystem
  Multiport Switch6 : MultiPortSwitch  Inputs=2  SaturateOnIntegerOverflow=on
  Multiport Switch7 : MultiPortSwitch  Inputs=2  SaturateOnIntegerOverflow=on
  Sw_ESP[0Off|1ABS|ESP] : Outport
  Sw_ASR[0Off|1On] : Outport  Port=2
  wires:
  Multiport Switch7/1 -> Sw_ESP[0Off|1ABS|ESP]/1
  Multiport Switch6/1 -> Sw_ASR[0Off|1On]/1
  Switches_ESP_User/1 -> Bus Selector2/1
  ECU_Commands[]/1 -> Maneuver/1(ECU_Commands[])
  Bus Selector2/1 -> Multiport Switch7/1, Multiport Switch6/1  "<Sw_ESP_Control_Mode[1ManSched|2Manual]>"
  Bus Selector2/2 -> Multiport Switch7/3  "<Sw_ESP[0Off|1ABS|2ESP]>"
  Bus Selector2/3 -> Multiport Switch6/3  "<SW_ASR[0Off|1On]>"
  Maneuver/1(Sw_ESP[0Off|1ABS|2ESP]) -> Multiport Switch7/2
  Maneuver/2(Sw_ASR0Off|1On]) -> Multiport Switch6/2
  Reset[0|1]/1 -> Maneuver/2(Reset[0|1])

== system ASM_Traffic_V2X_Complete_Model_2/MDL/SoftECU/OpenBrkHydModel ==

== system ASM_Traffic_V2X_Complete_Model_2/MDL/SoftECU/Soft_ECU_ACC ==
  Environment_Signals : Inport
  Vehicle_Signals : Inport  Port=2
  ASMSignalCollector : Subsystem
  Bus Selector2 : BusSelector  OutputSignals=Maneuver.UserSignals_Customized.ECU_Commands[]
  Bus Selector3 : BusSelector  OutputSignals=Environment.Driver.OutputSignals.Pos_AccPedal[%],Environment.Driver.OutputSignals.Pos_BrakePedal[%]
  Bus Selector4 : BusSelector  OutputSignals=VehicleDynamics.VehicleMovement.Velocities.Vehicle.Linear.v_Vehicle_CoG[x;y;z][km|h].v_x_Vehicle_CoG[km|h],VehicleDynamics.VehicleMovement.Velocities.Vehicle.Angular.w_Vehicle_CoG[x;y;z][deg|s].YawRate_Vehicle_CoG[deg|s],VehicleDynamics.Suspension.SuspensionFront.SuspensionKinematicsFront.Kinematics_Left.Position_Left.Pos_FL_Wheel[x;y;z][m],VehicleDynamics.Suspension.SuspensionFront.SuspensionKinematicsFront.Kinematics_Right.Position_Right.Pos_FR_Wheel[x;y;z][m]
  Bus Selector5 : BusSelector  OutputSignals=VehicleDynamics.Tire,VehicleDynamics.Aerodynamics.Coefficients.Cw_x[],Drivetrain.FinalDriveAssembly.i_FinalDrive[],Drivetrain.Transmission.ActiveTransmission.i_unsync_Trm[],VehicleDynamics.VehicleMovement.VehicleMassAndAdditionalLoads.m_TotalVehicle[kg],Environment.Road.Road_ASMVeh.Slope_Veh_Road[%],VehicleDynamics.VehicleMovement.Velocities.Vehicle.Linear.v_Vehicle_CoG[x;y;z][km|h].v_x_Vehicle_CoG[km|h],BasicEngine.EngineTorques.Trq_Fric_Engine[Nm]
  Bus Selector6 : BusSelector  OutputSignals=Traffic.Sensors.Object_Sensor_3D.Sensor_1_ACC.Dist_Object[m],Traffic.Sensors.Object_Sensor_3D.Sensor_1_ACC.v_Rel_Object[m|s],Traffic.Sensors.Object_Sensor_3D.Sensor_1_ACC.Angle_Hor_Object[deg],Maneuver.MdlControl.Reset_VehicleStates[0|1],Traffic.FellowMovement.s_Fellows_Ref_Scheduler[m],Traffic.FellowMovement.d_Total_Fellows_Road[m],Road.Road_ASMVeh.s_Veh_Road[m],Road.Road_ASMVeh.d_Total_Veh_Road[m],Traffic.Objects_Signals.FellowsGeometry.PosVec_MainPnt_Fellows[x;y;z][m],Traffic.Objects_Signals.FellowsGeometry.Size_Fellows[m].Length_Fellows[m],Traffic.Objects_Signals.FellowsGeometry.Size_Fellows[m].Width_Fellows[m],Traffic.Objects_Signals.FellowsGeometry.Size_Fellows[m].Height_Fellows[m],Traffic.Sensors.Object_Sensor_3D.Sensor_2_ACC.Object_ID[]
  Input_Selection : Subsystem
  Map_Inputs : Subsystem
  OUTPUT_INTERFACE_ACC : ASM_Traffic_lib/SoftECU/OUTPUT_INTERFACE_ACC  Tag=ASM_SUBCOMPONENT  ASMProperties=struct('Name','OUTPUT_INTERFACE_ACC','Version','3.0','Library','ASM_Traffic_lib')  ASMInstanceName=SoftECU_ACC  ASMInstanceID=1
  Rate Transition : RateTransition  Integrity=off  OutPortSampleTimeOpt=Inherit
  Rate Transition1 : RateTransition  Integrity=off  OutPortSampleTimeOpt=Inherit
  SOFT_ECU_ACC : ASM_Traffic_lib/SoftECU/SOFT_ECU_ACC  Tag=ASM_SUBCOMPONENT  Const_Kp_Dist_Ctrl=MDL.SoftECU.ACC.Const_Kp_Dist_Ctrl  Const_Ki_Dist_Ctrl=MDL.SoftECU.ACC.Const_Ki_Dist_Ctrl  Const_Kp_v_Ctrl=MDL.SoftECU.ACC.Const_Kp_v_Ctrl  Const_Ki_v_Ctrl=MDL.SoftECU.ACC.Const_Ki_v_Ctrl  Map_a_UpperLimit=MDL.SoftECU.ACC.Map_a_UpperLimit  Map_a_LowerLimit=MDL.SoftECU.ACC.Map_a_LowerLimit  Const_v_Threshold=MDL.SoftECU.ACC.Const_v_Threshold  Const_Dist_Threshold=MDL.SoftECU.ACC.Const_Dist_Threshold  Map_a_RisingRateMax=MDL.SoftECU.ACC.Map_a_RisingRateMax  Map_a_FallingRateMax=MDL.SoftECU.ACC.Map_a_FallingRateMax  Const_a_Max_AEB=MDL.SoftECU.ACC.Const_a_Max_AEB  Const_Response_Time_FCW=MDL.SoftECU.ACC.Const_Response_Time_FCW  Const_Dist_Min_Set=MDL.SoftECU.ACC.Const_Dist_Min_Set  Map_TTCThresholdAEB=MDL.SoftECU.ACC.Map_TTCThresholdAEB  StepSize=SIM.StepSize  ASMProperties=struct('Name','SOFT_ECU_ACC','Version','7.0','Library','ASM_Traffic_lib')  ASMInstanceName=SoftECU_ACC  ASMInstanceID=1
  Sw_ACC_Distance[s] : Constant  Value=2
  TARGET_SELECTION_ACC : ASM_Traffic_lib/SoftECU/TARGET_SELECTION_ACC  Tag=ASM_SUBCOMPONENT  Const_Dist_SafetyBound=MDL.SoftECU.ACC.Const_Dist_SafetyBound  Sw_LaneCrossingCheck=MDL.SoftECU.ACC.Sw_LaneCrossingCheck  StepSize=SIM.StepSize  ASMProperties=struct('Name','TARGET_SELECTION_ACC','Version','5.0','Library','ASM_Traffic_lib')  ASMInstanceName=SoftECU_ACC  ASMInstanceID=1
  Tire : Subsystem
  TrackWidthVehicle : Subsystem
  USER_INTERFACE_ACC : ASM_Traffic_lib/SoftECU/USER_INTERFACE_ACC  Tag=ASM_SUBCOMPONENT  Const_v_Step=MDL.SoftECU.ACC.Const_v_Step_CC  ASMProperties=struct('Name','USER_INTERFACE_ACC','Version','4.0','Library','ASM_Traffic_lib')  ASMInstanceName=SoftECU_ACC  ASMInstanceID=1
  hide_algebraic_loop : UnitDelay  SampleTime=-1
  hide_algebraic_loop1 : UnitDelay  SampleTime=-1
  "hide_algebraic_loop2 " : UnitDelay  SampleTime=-1
  ASMSignalBus : Outport
  Enable_Trq_Engine_ACC[0|1] : Outport  Port=2
  Trq_Request_Engine_ACC[Nm] : Outport  Port=3
  Enable_Trq_Brake_ACC[0|1] : Outport  Port=4
  Trq_Request_Brake_ACC[Nm] : Outport  Port=5
  tag scope: ASMBUS_SoftECU_ACC_Controller=global, ASMBUS_SoftECU_ACC_Interface=global, ASMBUS_SoftECU_ACC_Target_Selection=global, ASMBUS_SoftECU_ACC_User_Interface=global
  wires:
  Rate Transition1/1 -> TARGET_SELECTION_ACC/8
  Input_Selection/1(PosVec_MainPnt_Out) -> TARGET_SELECTION_ACC/12
  Bus Selector6/9 -> Input_Selection/1(PosVec_MainPnt_In)  "<PosVec_MainPnt_Fellows[x;y;z][m]>"
  Bus Selector6/12 -> TARGET_SELECTION_ACC/15  "<Height_Fellows[m]>"
  Bus Selector6/11 -> TARGET_SELECTION_ACC/14  "<Width_Fellows[m]>"
  Bus Selector6/10 -> TARGET_SELECTION_ACC/13  "<Length_Fellows[m]>"
  TARGET_SELECTION_ACC/6 -> SOFT_ECU_ACC/6
  TARGET_SELECTION_ACC/5 -> SOFT_ECU_ACC/5
  Bus Selector6/13 -> TARGET_SELECTION_ACC/16  "<Object_ID[]>"
  Bus Selector6/8 -> TARGET_SELECTION_ACC/11  "<d_Total_Veh_Road[m]>"
  Bus Selector6/7 -> TARGET_SELECTION_ACC/10  "<s_Veh_Road[m]>"
  Bus Selector6/5 -> Rate Transition1/1  "<s_Fellows_Ref_Scheduler[m]>"
  Bus Selector6/6 -> TARGET_SELECTION_ACC/9  "<d_Total_Fellows_Road[m]>"
  Bus Selector6/4 -> TARGET_SELECTION_ACC/7, USER_INTERFACE_ACC/11, Map_Inputs/1(Reset[0|1])  "<Reset_VehicleStates[0|1]>"
  Bus Selector6/3 -> TARGET_SELECTION_ACC/6  "<Angle_Hor_Object[deg]>"
  Bus Selector6/2 -> TARGET_SELECTION_ACC/5  "<v_Rel_Object[m|s]>"
  Bus Selector6/1 -> TARGET_SELECTION_ACC/4  "<Dist_Object[m]>"
  TrackWidthVehicle/1(TrackWidth_Vehicle[m]) -> TARGET_SELECTION_ACC/3
  Bus Selector4/4 -> TrackWidthVehicle/2(Pos_FR_Wheel[x;y;z][m])  "<Pos_FR_Wheel[x;y;z][m]>"
  Bus Selector4/3 -> TrackWidthVehicle/1(Pos_FL_Wheel[x;y;z][m])  "<Pos_FL_Wheel[x;y;z][m]>"
  Bus Selector3/2 -> USER_INTERFACE_ACC/3  "<Pos_BrakePedal[%]>"
  Bus Selector3/1 -> USER_INTERFACE_ACC/2  "<Pos_AccPedal[%]>"
  hide_algebraic_loop/1 -> OUTPUT_INTERFACE_ACC/1
  "hide_algebraic_loop2 "/1 -> Enable_Trq_Brake_ACC[0|1]/1, OUTPUT_INTERFACE_ACC/12
  hide_algebraic_loop1/1 -> Enable_Trq_Engine_ACC[0|1]/1, OUTPUT_INTERFACE_ACC/11
  SOFT_ECU_ACC/4 -> "hide_algebraic_loop2 "/1
  SOFT_ECU_ACC/3 -> hide_algebraic_loop1/1
  Rate Transition/1 -> SOFT_ECU_ACC/2
  Map_Inputs/8(Sw_ACC_BrakeMode[1Comfort|2AEBOnly|3AEBOff]) -> SOFT_ECU_ACC/9
  TARGET_SELECTION_ACC/2 -> Rate Transition/1
  TARGET_SELECTION_ACC/3 -> SOFT_ECU_ACC/3
  TARGET_SELECTION_ACC/4 -> SOFT_ECU_ACC/4
  USER_INTERFACE_ACC/3 -> SOFT_ECU_ACC/8
  Sw_ACC_Distance[s]/1 -> SOFT_ECU_ACC/10
  Bus Selector2/1 -> Map_Inputs/3(ECU_Commands[])  "<ECU_Commands[]>"
  [ASMBUS_Environment] -> Bus Selector2/1
  [TAG_SoftECU_Switches_ACC] -> Map_Inputs/2(Switches_ACC_User)
  Map_Inputs/7(Sw_ACC_Speed_Decrease[0Off|1On]) -> USER_INTERFACE_ACC/10
  Map_Inputs/6(Sw_ACC_Speed_Increase[0Off|1On]) -> USER_INTERFACE_ACC/9
  Map_Inputs/5(Sw_ACC_Speed_Set[0Off|1On]) -> USER_INTERFACE_ACC/8
  Map_Inputs/4(Sw_ACC_Resume[0Off|1On]) -> USER_INTERFACE_ACC/7
  Map_Inputs/3(Sw_ACC_Cancel[0Off|1On]) -> USER_INTERFACE_ACC/6
  Map_Inputs/2(Sw_ACC_Off[0Off|1On]) -> USER_INTERFACE_ACC/5
  Map_Inputs/1(Sw_ACC_On[0Off|1On]) -> USER_INTERFACE_ACC/4
  USER_INTERFACE_ACC/1 -> [ASMBUS_SoftECU_ACC_User_Interface]
  Bus Selector5/3 -> OUTPUT_INTERFACE_ACC/5  "<i_FinalDrive[]>"
  TARGET_SELECTION_ACC/1 -> [ASMBUS_SoftECU_ACC_Target_Selection]
  SOFT_ECU_ACC/2 -> hide_algebraic_loop/1
  Bus Selector4/2 -> TARGET_SELECTION_ACC/1  "<YawRate_Vehicle_CoG[deg|s]>"
  USER_INTERFACE_ACC/2 -> SOFT_ECU_ACC/7
  Bus Selector5/5 -> OUTPUT_INTERFACE_ACC/7  "<m_TotalVehicle[kg]>"
  Bus Selector5/4 -> OUTPUT_INTERFACE_ACC/6  "<i_unsync_Trm[]>"
  OUTPUT_INTERFACE_ACC/1 -> [ASMBUS_SoftECU_ACC_Interface]
  OUTPUT_INTERFACE_ACC/2 -> Trq_Request_Brake_ACC[Nm]/1
  OUTPUT_INTERFACE_ACC/3 -> Trq_Request_Engine_ACC[Nm]/1
  Bus Selector5/8 -> OUTPUT_INTERFACE_ACC/10  "<Trq_Fric_Engine[Nm]>"
  Bus Selector5/7 -> OUTPUT_INTERFACE_ACC/9  "<v_x_Vehicle_CoG[km|h]>"
  Bus Selector5/6 -> OUTPUT_INTERFACE_ACC/8  "<Slope_Veh_Road[%]>"
  Bus Selector5/2 -> OUTPUT_INTERFACE_ACC/4  "<Cw_x[]>"
  Bus Selector5/1 -> Tire/1(Tire)  "<Tire>"
  Tire/2(Coef_RollingRes_Mean[]) -> OUTPUT_INTERFACE_ACC/3
  Tire/1(r_Dyn_Tire_Mean[m]) -> OUTPUT_INTERFACE_ACC/2
  ASMSignalCollector/1(ASMSignalBus) -> ASMSignalBus/1
  Bus Selector4/1 -> SOFT_ECU_ACC/1, TARGET_SELECTION_ACC/2, USER_INTERFACE_ACC/1  "<v_x_Vehicle_CoG[km|h]>"
  SOFT_ECU_ACC/1 -> [ASMBUS_SoftECU_ACC_Controller]
  Environment_Signals/1 -> Bus Selector6/1
  Vehicle_Signals/1 -> Bus Selector5/1, Bus Selector3/1, Bus Selector4/1

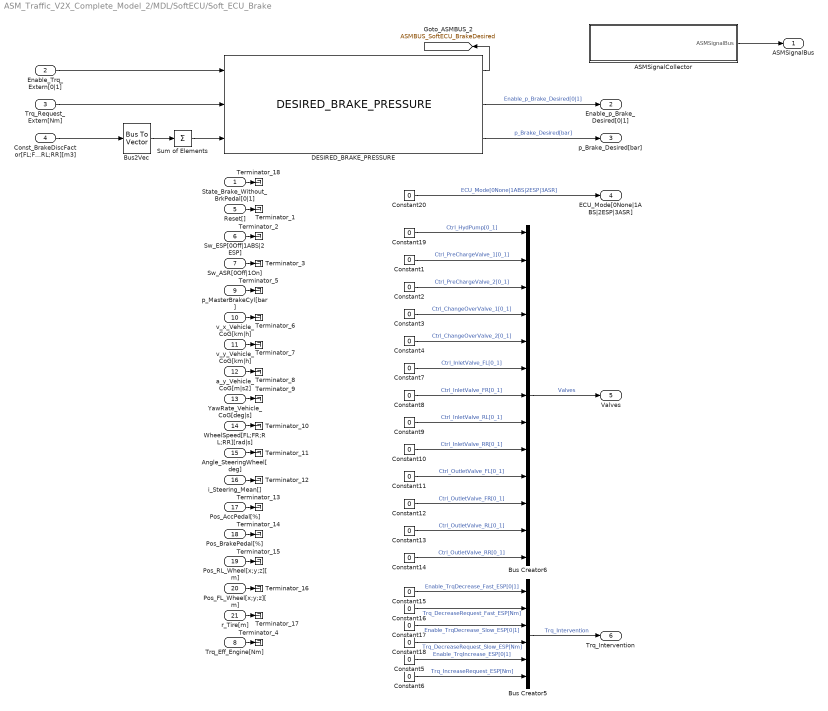
== system ASM_Traffic_V2X_Complete_Model_2/MDL/SoftECU/Soft_ECU_Brake ==
  State_Brake_Without_BrkPedal[0|1] : Inport
  Enable_Trq_Extern[0|1] : Inport  Port=2
  Trq_Request_Extern[Nm] : Inport  Port=3
  Const_BrakeDiscFactor[FL;FR;RL;RR][m3] : Inport  Port=4
  Reset[] : Inport  Port=5
  Sw_ESP[0Off|1ABS|2ESP] : Inport  Port=6
  Sw_ASR[0Off|1On] : Inport  Port=7
  Trq_Eff_Engine[Nm] : Inport  Port=8
  p_MasterBrakeCyl[bar] : Inport  Port=9
  v_x_Vehicle_CoG[km|h] : Inport  Port=10
  v_y_Vehicle_CoG[km|h] : Inport  Port=11
  a_y_Vehicle_CoG[m|s2] : Inport  Port=12
  YawRate_Vehicle_CoG[deg|s] : Inport  Port=13
  WheelSpeed[FL;FR;RL;RR][rad|s] : Inport  Port=14
  Angle_SteeringWheel[deg] : Inport  Port=15
  i_Steering_Mean[] : Inport  Port=16
  Pos_AccPedal[%] : Inport  Port=17
  Pos_BrakePedal[%] : Inport  Port=18
  Pos_RL_Wheel[x;y;z][m] : Inport  Port=19
  Pos_FL_Wheel[x;y;z][m] : Inport  Port=20
  r_Tire[m] : Inport  Port=21
  ASMSignalCollector : Subsystem
  Bus Creator5 : BusCreator  Inputs=6
  Bus Creator6 : BusCreator  Inputs=13
  Bus2Vec : BusToVector
  Constant{1..20} (20 alike) : Constant  Value=0
  DESIRED_BRAKE_PRESSURE : ASM_BrakeHydraulics_lib/SoftECU/DESIRED_BRAKE_PRESSURE  Tag=ASM_SUBCOMPONENT  ASMProperties=struct('Name','DESIRED_BRAKE_PRESSURE','Version','2.0','Library','ASM_BrakeHydraulics_lib')  ASMInstanceName=desired_brake_pressure  ASMInstanceID=1
  Sum of Elements : Sum  Inputs=+
  Terminator_{1..18} (18 alike) : Terminator
  ASMSignalBus : Outport
  Enable_p_Brake_Desired[0|1] : Outport  Port=2
  p_Brake_Desired[bar] : Outport  Port=3
  ECU_Mode[0None|1ABS|2ESP|3ASR] : Outport  Port=4
  Valves : Outport  Port=5
  Trq_Intervention : Outport  Port=6
  tag scope: ASMBUS_SoftECU_BrakeDesired=global
  wires:
  Sum of Elements/1 -> DESIRED_BRAKE_PRESSURE/3
  DESIRED_BRAKE_PRESSURE/1 -> [ASMBUS_SoftECU_BrakeDesired]
  Constant15/1 -> Bus Creator5/1  "Enable_TrqDecrease_Fast_ESP[0|1]"
  Constant17/1 -> Bus Creator5/3  "Enable_TrqDecrease_Slow_ESP[0|1]"
  Constant18/1 -> Bus Creator5/4  "Trq_DecreaseRequest_Slow_ESP[Nm]"
  Constant5/1 -> Bus Creator5/5  "Enable_TrqIncrease_ESP[0|1]"
  Constant6/1 -> Bus Creator5/6  "Trq_IncreaseRequest_ESP[Nm]"
  Constant7/1 -> Bus Creator6/6  "Ctrl_InletValve_FL[0_1]"
  Constant8/1 -> Bus Creator6/7  "Ctrl_InletValve_FR[0_1]"
  Constant9/1 -> Bus Creator6/8  "Ctrl_InletValve_RL[0_1]"
  Constant10/1 -> Bus Creator6/9  "Ctrl_InletValve_RR[0_1]"
  Constant11/1 -> Bus Creator6/10  "Ctrl_OutletValve_FL[0_1]"
  Constant12/1 -> Bus Creator6/11  "Ctrl_OutletValve_FR[0_1]"
  Constant13/1 -> Bus Creator6/12  "Ctrl_OutletValve_RL[0_1]"
  Constant14/1 -> Bus Creator6/13  "Ctrl_OutletValve_RR[0_1]"
  Constant1/1 -> Bus Creator6/2  "Ctrl_PreChargeValve_1[0_1]"
  Constant2/1 -> Bus Creator6/3  "Ctrl_PreChargeValve_2[0_1]"
  Constant3/1 -> Bus Creator6/4  "Ctrl_ChangeOverValve_1[0_1]"
  Constant4/1 -> Bus Creator6/5  "Ctrl_ChangeOverValve_2[0_1]"
  DESIRED_BRAKE_PRESSURE/2 -> Enable_p_Brake_Desired[0|1]/1  "Enable_p_Brake_Desired[0|1]"
  DESIRED_BRAKE_PRESSURE/3 -> p_Brake_Desired[bar]/1  "p_Brake_Desired[bar]"
  Enable_Trq_Extern[0|1]/1 -> DESIRED_BRAKE_PRESSURE/1
  Bus Creator5/1 -> Trq_Intervention/1  "Trq_Intervention"
  Trq_Request_Extern[Nm]/1 -> DESIRED_BRAKE_PRESSURE/2
  Bus Creator6/1 -> Valves/1  "Valves"
  Const_BrakeDiscFactor[FL;FR;RL;RR][m3]/1 -> Bus2Vec/1
  Bus2Vec/1 -> Sum of Elements/1
  Constant16/1 -> Bus Creator5/2  "Trq_DecreaseRequest_Fast_ESP[Nm]"
  Constant19/1 -> Bus Creator6/1  "Ctrl_HydPump[0_1]"
  Constant20/1 -> ECU_Mode[0None|1ABS|2ESP|3ASR]/1  "ECU_Mode[0None|1ABS|2ESP|3ASR]"
  Reset[]/1 -> Terminator_1/1
  Sw_ESP[0Off|1ABS|2ESP]/1 -> Terminator_2/1
  Sw_ASR[0Off|1On]/1 -> Terminator_3/1
  Trq_Eff_Engine[Nm]/1 -> Terminator_4/1
  p_MasterBrakeCyl[bar]/1 -> Terminator_5/1
  v_x_Vehicle_CoG[km|h]/1 -> Terminator_6/1
  v_y_Vehicle_CoG[km|h]/1 -> Terminator_7/1
  a_y_Vehicle_CoG[m|s2]/1 -> Terminator_8/1
  YawRate_Vehicle_CoG[deg|s]/1 -> Terminator_9/1
  WheelSpeed[FL;FR;RL;RR][rad|s]/1 -> Terminator_10/1
  Angle_SteeringWheel[deg]/1 -> Terminator_11/1
  i_Steering_Mean[]/1 -> Terminator_12/1
  Pos_AccPedal[%]/1 -> Terminator_13/1
  Pos_BrakePedal[%]/1 -> Terminator_14/1
  Pos_RL_Wheel[x;y;z][m]/1 -> Terminator_15/1
  Pos_FL_Wheel[x;y;z][m]/1 -> Terminator_16/1
  r_Tire[m]/1 -> Terminator_17/1
  ASMSignalCollector/1(ASMSignalBus) -> ASMSignalBus/1
  State_Brake_Without_BrkPedal[0|1]/1 -> Terminator_18/1
